simulink model "Model_matlab"  (Simulink 10.0)
settings: Solver=VariableStepAuto  StartTime=0.0  StopTime=30  RelTol=1e-3
values from neighbouring files (symbols this model uses):
  J = 0.03    [parametry.m]
  k = 1.52    [parametry.m]
  La = 0.035    [parametry.m]
  R = 4.6    [parametry.m]
settings Model: Creator=Lenovo  LastModifiedBy=szymo
settings DataIOCC: SaveFormat=Dataset  ReturnWorkspaceOutputs=on
settings OptimizationCC: LifeSpan=auto
settings DebuggingCC: UnderspecifiedInitializationDetection=Simplified  MergeDetectMultiDrivingBlocksExec=error  SFUnexpectedBacktrackingDiag=error  SFNoUnconditionalDefaultTransitionDiag=error  SFExecutionAtInitializationDiag=warning  ArithmeticOperatorsInVariantConditions=error
settings HardwareCC: ProdBitPerPointer=64  ProdBitPerSizeT=64  ProdBitPerPtrDiffT=64  ProdLargestAtomicFloat=Float  ProdIntDivRoundTo=Zero  ProdEndianess=LittleEndian  ProdWordSize=64  ProdHWDeviceType=Intel->x86-64 (Windows64)
settings ModelReferenceCC: PropagateSignalLabelsOutOfModel=on
settings SFSimCC: SimUseLocalCustomCode=on  CustomCodeUndefinedFunction=FilterOut
settings RTWCC: RTWUseLocalCustomCode=on
settings CodeAppCC: StateflowObjectComments=off
settings GRTTargetCC: TargetLangStandard=C99 (ISO)  CombineOutputUpdateFcns=on  GRTInterface=off
settings ConfigComp: CovMetricSettings=dwe  CovHtmlReporting=off  CovSaveCumulativeToWorkspaceVar=off  CovSaveSingleToWorkspaceVar=off

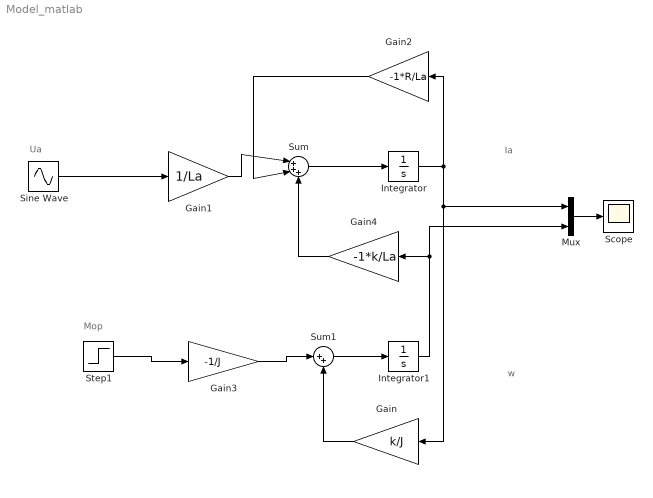
== system Model_matlab ==
  note: Ua
  note: Mop
  note: w
  note: Ia
  Gain : Gain  Gain=k/J
  Gain1 : Gain  Gain=1/La
  Gain2 : Gain  Gain=-1*R/La
  Gain3 : Gain  Gain=-1/J
  Gain4 : Gain  Gain=-1*k/La
  Integrator : Integrator
  Integrator1 : Integrator
  Mux : Mux  Inputs=2
  Scope : Scope
  Sine Wave : Sin  Amplitude=230  Frequency=50  SampleTime=0
  Step1 : Step  SampleTime=0
  Sum : Sum  Inputs=|+++
  Sum1 : Sum  Inputs=|++
  wires:
  Gain1/1 -> Sum/1
  Sum/1 -> Integrator/1
  Integrator/1 -> Mux/1, Gain/1, Gain2/1
  Gain2/1 -> Sum/2
  Gain3/1 -> Sum1/1
  Sum1/1 -> Integrator1/1
  Integrator1/1 -> Mux/2, Gain4/1
  Gain4/1 -> Sum/3
  Gain/1 -> Sum1/2
  Sine Wave/1 -> Gain1/1
  Step1/1 -> Gain3/1
  Mux/1 -> Scope/1
